simulink model "P1_COMPARATIVA"  (R2016b)
settings: Solver=ode4  StartTime=0.0  StopTime=100  FixedStep=dt  RelTol=1e-3  EnableMultiTasking=on
values from neighbouring files (symbols this model uses):
  Ap = [-2*sqrt(B*Fpnom)/m 1/m 0 0 ... (first row only)    [Ejercicio1.m]
  B = 0.162    [Ejercicio1.m]
  Bp = [0 Kt/taup 0 0]'    [Ejercicio1.m]
  COnom = Fpnom/Kt    (= 5)    [Ejercicio1.m]
  Cp = [0 0 0 1]    [Ejercicio1.m]
  Dp = 0    [Ejercicio1.m]
  Fpdotlim = [-1 1]*16e3/5    [Ejercicio1.m]
  Fplim = [0 1]*16e3    [Ejercicio1.m]
  Fpnom = 8e3    (= 8000)    [Ejercicio1.m]
  Km = 10/300    (= 0.0333333333333)    [Ejercicio1.m]
  Kt = 16e3/10    (= 1600)    [Ejercicio1.m]
  m = 400    [Ejercicio1.m]
  tauf = 0.02    [Ejercicio1.m]
  taum = 0.1    [Ejercicio1.m]
  taup = 1    [Ejercicio1.m]
  Vmfnom = Vmnom    (= 7.40740740741)    [Ejercicio1.m]
  Vmlim = [0 10]    [Ejercicio1.m]
  Vmnom = Vnom*Km    (= 7.40740740741)    [Ejercicio1.m]
  Vnom = 800*10/36    (= 222.222222222)    [Ejercicio1.m]
settings Model: Creator=Jairo  LastModifiedBy=elena
settings DataIOCC: LimitDataPoints=on  SaveFormat=Array
settings OptimizationCC: LifeSpan=inf
settings DebuggingCC: SolverPrmCheckMsg=warning  SFUnexpectedBacktrackingDiag=warning  SFNoUnconditionalDefaultTransitionDiag=warning  SFExecutionAtInitializationDiag=none
settings HardwareCC: ProdBitPerPointer=32  ProdBitPerSizeT=32  ProdBitPerPtrDiffT=32  ProdLargestAtomicFloat=None  ProdIntDivRoundTo=Undefined  ProdEndianess=Unspecified  ProdWordSize=32  ProdHWDeviceType=32-bit Generic
settings ModelReferenceCC: PropagateSignalLabelsOutOfModel=off
settings GRTTargetCC: TargetLangStandard=C89/C90 (ANSI)  GeneratePreprocessorConditionals=Disable all
settings ConfigComp: CovMetricSettings=dw  CovHtmlReporting=on  CovSaveCumulativeToWorkspaceVar=on  CovSaveSingleToWorkspaceVar=on  CovExternalEMLEnable=off  CovSFcnEnable=off

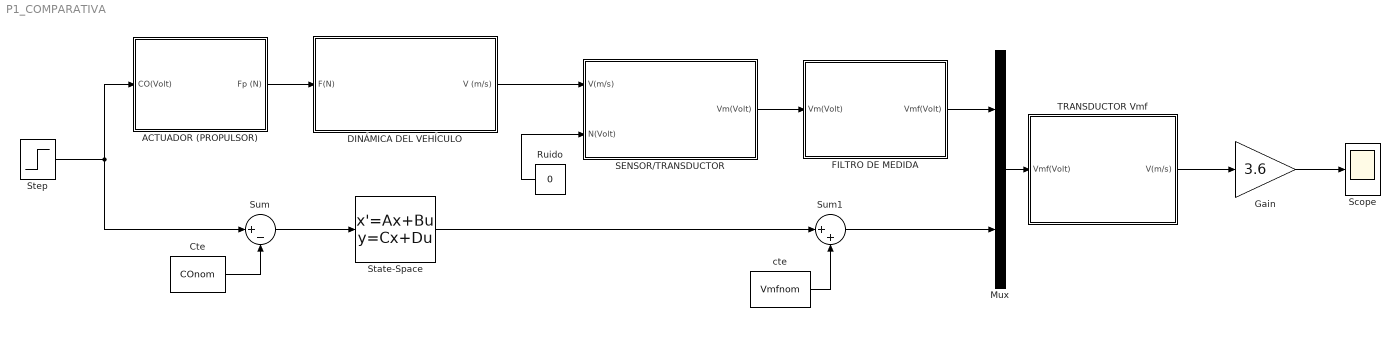
== system P1_COMPARATIVA ==
  ACTUADOR (PROPULSOR) : Subsystem
  Cte : Constant  Value=COnom
  DINÁMICA DEL VEHÍCULO : Subsystem
  FILTRO DE MEDIDA : Subsystem
  Gain : Gain  Gain=3.6
  Mux : Mux  Inputs=2
  Ruido : Constant  Value=0
  SENSOR/TRANSDUCTOR : Subsystem
  Scope : Scope
  State-Space : StateSpace  A=Ap  B=Bp  C=Cp  D=Dp  X0=[0 0 0 0]
  Step : Step  Time=10  Before=COnom  After=COnom+1  SampleTime=0
  Sum : Sum  Inputs=|+-
  Sum1 : Sum  Inputs=|++
  TRANSDUCTOR Vmf : Subsystem
  cte : Constant  Value=Vmfnom
  wires:
  Gain/1 -> Scope/1
  Ruido/1 -> SENSOR/TRANSDUCTOR/2(N(Volt))
  ACTUADOR (PROPULSOR)/1(Fp (N)) -> DINÁMICA DEL VEHÍCULO/1(F(N))
  DINÁMICA DEL VEHÍCULO/1(V (m/s)) -> SENSOR/TRANSDUCTOR/1(V(m/s))
  SENSOR/TRANSDUCTOR/1(Vm(Volt)) -> FILTRO DE MEDIDA/1(Vm(Volt))
  Mux/1 -> TRANSDUCTOR Vmf/1(Vmf(Volt))
  TRANSDUCTOR Vmf/1(V(m/s)) -> Gain/1
  Step/1 -> ACTUADOR (PROPULSOR)/1(CO(Volt)), Sum/1
  Cte/1 -> Sum/2
  Sum/1 -> State-Space/1
  State-Space/1 -> Sum1/1
  cte/1 -> Sum1/2
  Sum1/1 -> Mux/2
  FILTRO DE MEDIDA/1(Vmf(Volt)) -> Mux/1

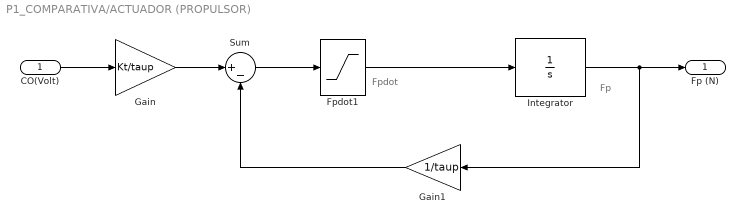
== system P1_COMPARATIVA/ACTUADOR (PROPULSOR) ==
  note: Fp
  note: Fpdot
  CO(Volt) : Inport
  Fpdot1 : Saturate  UpperLimit=Fpdotlim(2)  LowerLimit=Fpdotlim(1)
  Gain : Gain  Gain=Kt/taup
  Gain1 : Gain  Gain=1/taup
  Integrator : Integrator  InitialCondition=Fpnom  LimitOutput=on  UpperSaturationLimit=Fplim(2)  LowerSaturationLimit=Fplim(1)
  Sum : Sum  Inputs=|+-
  Fp (N) : Outport
  wires:
  CO(Volt)/1 -> Gain/1
  Gain/1 -> Sum/1
  Sum/1 -> Fpdot1/1
  Fpdot1/1 -> Integrator/1
  Integrator/1 -> Fp (N)/1, Gain1/1
  Gain1/1 -> Sum/2

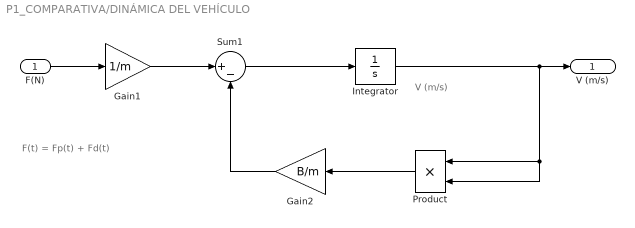
== system P1_COMPARATIVA/DINÁMICA DEL VEHÍCULO ==
  note: F(t) = Fp(t) + Fd(t)
  note: V (m/s)
  F(N) : Inport
  Gain1 : Gain  Gain=1/m
  Gain2 : Gain  Gain=B/m
  Integrator : Integrator  InitialCondition=Vnom
  Product : Product
  Sum1 : Sum  Inputs=|+-
  V (m/s) : Outport
  wires:
  F(N)/1 -> Gain1/1
  Gain1/1 -> Sum1/1
  Sum1/1 -> Integrator/1
  Gain2/1 -> Sum1/2
  Integrator/1 -> V (m/s)/1, Product/2, Product/1
  Product/1 -> Gain2/1

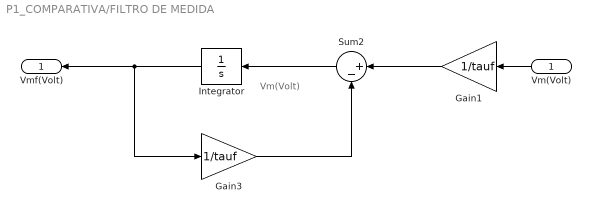
== system P1_COMPARATIVA/FILTRO DE MEDIDA ==
  note: Vm(Volt)
  Vm(Volt) : Inport
  Gain1 : Gain  Gain=1/tauf
  Gain3 : Gain  Gain=1/tauf
  Integrator : Integrator  InitialCondition=Vmfnom
  Sum2 : Sum  Inputs=|+-
  Vmf(Volt) : Outport
  wires:
  Vm(Volt)/1 -> Gain1/1
  Gain1/1 -> Sum2/1
  Sum2/1 -> Integrator/1
  Gain3/1 -> Sum2/2
  Integrator/1 -> Vmf(Volt)/1, Gain3/1

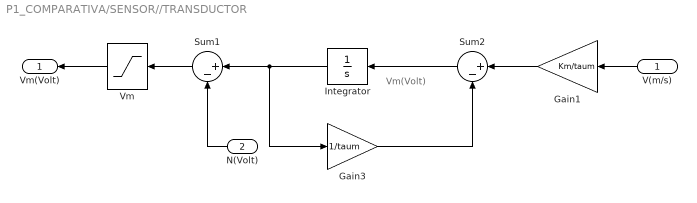
== system P1_COMPARATIVA/SENSOR//TRANSDUCTOR ==
  note: Vm(Volt)
  V(m/s) : Inport
  N(Volt) : Inport  Port=2
  Gain1 : Gain  Gain=Km/taum
  Gain3 : Gain  Gain=1/taum
  Integrator : Integrator  InitialCondition=Vmnom
  Sum1 : Sum  Inputs=|+-
  Sum2 : Sum  Inputs=|+-
  Vm : Saturate  UpperLimit=Vmlim(2)  LowerLimit=Vmlim(1)
  Vm(Volt) : Outport
  wires:
  V(m/s)/1 -> Gain1/1
  Gain1/1 -> Sum2/1
  Sum2/1 -> Integrator/1
  Integrator/1 -> Gain3/1, Sum1/1
  N(Volt)/1 -> Sum1/2
  Gain3/1 -> Sum2/2
  Sum1/1 -> Vm/1
  Vm/1 -> Vm(Volt)/1

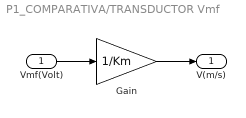
== system P1_COMPARATIVA/TRANSDUCTOR Vmf ==
  Vmf(Volt) : Inport
  Gain : Gain  Gain=1/Km  SaturateOnIntegerOverflow=on  OutDataTypeStr=Inherit: Same as input  ParamDataTypeStr=Inherit: Same as input
  V(m/s) : Outport
  wires:
  Vmf(Volt)/1 -> Gain/1
  Gain/1 -> V(m/s)/1
